simulink model "DigitalSignalSendingReceiving1"  (R2023b)
settings: Solver=FixedStepAuto  StartTime=0.0  StopTime=Inf  FixedStep=0.001  RelTol=1e-3
PostLoadFcn:
  | if any(exist('dsrtsu_mdlpostloadfcn', 'file') ~= 0), dsrtsu_mdlpostloadfcn('Execute', bdroot); end
InitFcn:
  | , if any(exist('rtifpga_mdlclblib', 'file') ~= 0), rtifpga_mdlclblib('Init', bdroot); end,
  | , if any(exist('dsmpb_private', 'file') ~= 0), dsmpb_private('dsmpb_mdlclblib', 'Init', bdroot); end,
libraries: dsmpblib x5
PreSaveFcn:
  | , if any(exist('dsmpb_private', 'file') ~= 0), dsmpb_private('dsmpb_mdlclblib', 'PreSave', bdroot); end,
CloseFcn:
  | , if any(exist('dsmpb_private', 'file') ~= 0), dsmpb_private('dsmpb_mdlclblib', 'Close', bdroot); end,
settings Model: DSRTSU_INTERNAL_RTIFPGA=210  DSRTSU_INTERNAL_RTISTBM_VER=23.2  DSMPB_ID_DATA={'1',struct('BlockId','509f4544-4437-4c2c-aedf-9c234d46aa93','SignalIds',{{'4a51c788-ee25-4617-bb29-856017da9ae4'}}),'12',struct('BlockId','d760b032-a650-4213-93d1-07351a748fbc','SignalIds',{{'2642401f-ce84-4f9c-bed9-38ea9fa046b2'}}),'14',struct('BlockId','326f3eb7-2503-4153-b75d-1cc4d2a57b45','SignalIds',{{'f48305e4-e0d8-49ed-b391-47f7934351d1','c31b1b5c-9715-44c6-b961-3146ac445240'}}),'7',struct('BlockId','6ff17c6b-b230-4bb3-82ba-89d1bfad999e','SignalIds',{{'01d15d83-bc53-4738-ad86-dfc1fef8a5b0'}}),'9',struct('BlockId','a7c6afe6-f4cc-4154-9fd1-22d7934362d7','SignalIds',{{'3544d482-4545-4c9f-bf36-a4984100c31b'}})}  Creator=MURTI  LastModifiedBy=MURTI
settings OptimizationCC: BlockReduction=off  ConditionallyExecuteInputs=off  OptimizeBlockIOStorage=off  BufferReuse=off
settings DebuggingCC: TasksWithSamePriorityMsg=none
settings HardwareCC: ProdBitPerLong=64  ProdLargestAtomicInteger=Integer  ProdWordSize=32  ProdLongLongMode=on  ProdHWDeviceType=Custom Processor->Custom
settings ModelReferenceCC: EnableParallelModelReferenceBuilds=on
settings RTWCC: Description=dSPACE Target DSRT - Generates SIC files for import by ConfigurationDesk and VEOS. Provides code generation for Simulink models imported in ConfigurationDesk.  SystemTargetFile=dsrt.tlc  GenCodeOnly=on  MakeCommand=make_dsrt  TemplateMakefile=dsrt_default_tmf  RTWVerbose=off
settings STFCustomTargetCC: ParMdlRefBuildCompliant=on  SystemTargetFile=dsrt.tlc
settings GRTTargetCC: CompOptLevelCompliant=off  ConcurrentExecutionCompliant=off  CombineOutputUpdateFcns=off  MatFileLogging=off  CPPClassGenCompliant=off  UseToolchainInfoCompliant=off

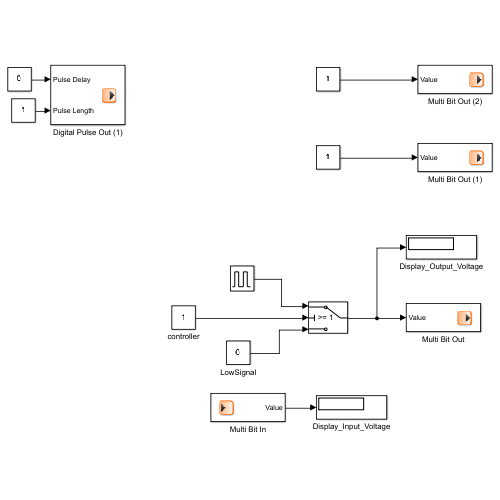
[thumbnail: Simulink's stored preview of the top-level diagram]
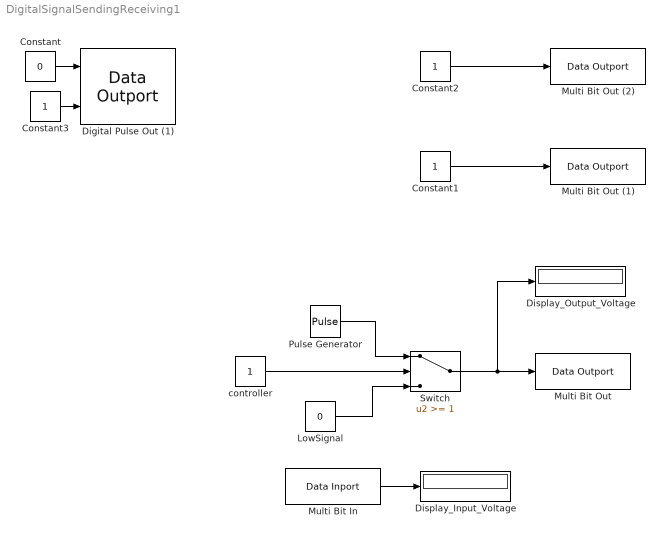
== system DigitalSignalSendingReceiving1 ==
  Constant : Constant  Value=0
  Constant1 : Constant
  Constant2 : Constant
  Constant3 : Constant
  Digital Pulse Out (1) : dsmpblib/Data Outport  Priority=-10000
      settings: SourceProductName=dSPACE Model Interface Package for Simulink (MIPS)
  Display_Input_Voltage : Display
  Display_Output_Voltage : Display
  LowSignal : Constant  Value=0
  Multi Bit In : dsmpblib/Data Inport  Priority=10000
      settings: SourceProductName=dSPACE Model Interface Package for Simulink (MIPS)
  Multi Bit Out : dsmpblib/Data Outport  Priority=-10000
      settings: SourceProductName=dSPACE Model Interface Package for Simulink (MIPS)
  Multi Bit Out (1) : dsmpblib/Data Outport  Priority=-10000
      settings: SourceProductName=dSPACE Model Interface Package for Simulink (MIPS)
  Multi Bit Out (2) : dsmpblib/Data Outport  Priority=-10000
      settings: SourceProductName=dSPACE Model Interface Package for Simulink (MIPS)
  Pulse Generator : DiscretePulseGenerator  PulseType=Time based  Period=10  PulseWidth=50
  Switch : Switch  Threshold=1  SaturateOnIntegerOverflow=off  InputSameDT=off
  controller : Constant
  wires:
  Pulse Generator/1 -> Switch/1
  controller/1 -> Switch/2
  LowSignal/1 -> Switch/3
  Switch/1 -> Display_Output_Voltage/1, Multi Bit Out/1
  Multi Bit In/1 -> Display_Input_Voltage/1
  Constant1/1 -> Multi Bit Out (1)/1
  Constant2/1 -> Multi Bit Out (2)/1
  Constant/1 -> Digital Pulse Out (1)/1
  Constant3/1 -> Digital Pulse Out (1)/2
